simulink model "model_FOPTD_DMD_5SensorScenario_v1"  (R2021b)
settings: Solver=FixedStepAuto  StartTime=0.0  StopTime=20  FixedStep=TsSystem  MaxStep=0.01  RelTol=1e-3
values from neighbouring files (symbols this model uses):
  da = 0    [runSimulation_v1.m]
  ds = numSim    [runSimulation_v1.m]
  K = 1    [runSimulation_v1.m]
  Ka = 0    [runSimulation_v1.m]
  Ks = 0    [runSimulation_v1.m]
  L = 1    [runSimulation_v1.m]
  T = 0.1    [runSimulation_v1.m]
  TsSystem = 0.01    [runSimulation_v1.m]
libraries: simulink x2, slpidlib x1
settings Model: Creator=ahmet  LastModifiedBy=ahmet
settings SolverCC: AlgebraicLoopSolver=TrustRegion
settings DebuggingCC: SFMachineParentedDataDiag=warning

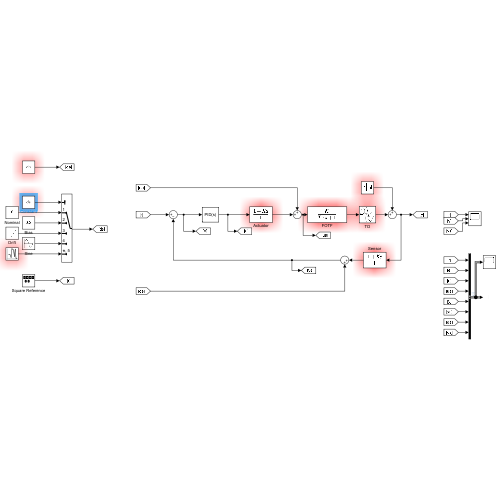
[thumbnail: Simulink's stored preview of the top-level diagram]
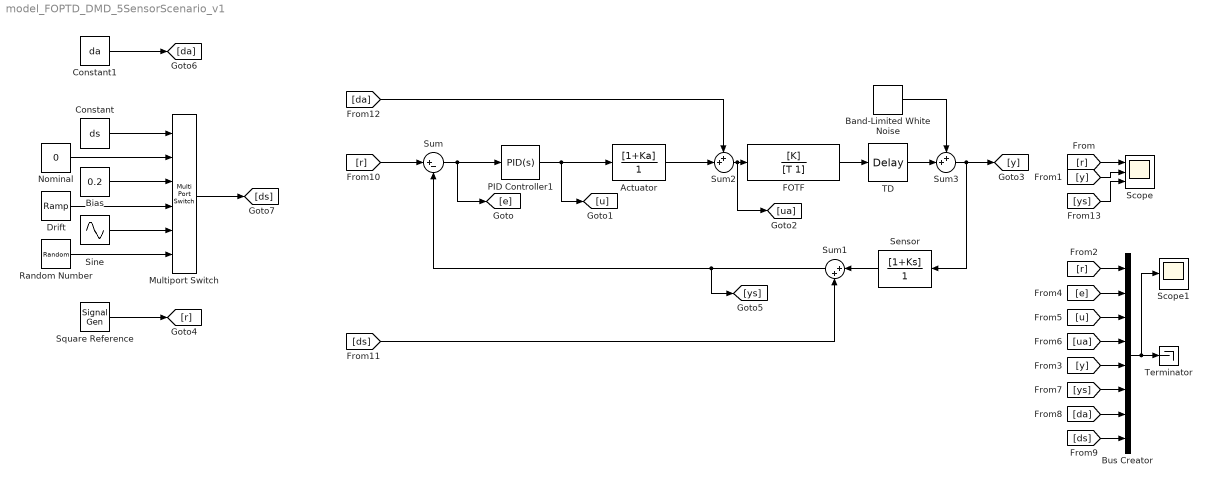
== system model_FOPTD_DMD_5SensorScenario_v1 ==
  Actuator : TransferFcn  Numerator=[1+Ka]  Denominator=[1]
  Band-Limited White Noise : simulink/Sources/Band-Limited White Noise  Cov=[1e-3*TsSystem]  Ts=TsSystem  seed=[23412+randi([-1000 1000],1,1)]
  Bias : Constant  Value=0.2
  Bus Creator : BusCreator  Inputs=8
  Constant : Constant  Value=ds
  Constant1 : Constant  Value=da
  Drift : simulink/Sources/Ramp  slope=1/10  start=0  InitialOutput=0
  FOTF : TransferFcn  Numerator=[K]  Denominator=[T 1]
  Multiport Switch : MultiPortSwitch  Inputs=5
  Nominal : Constant  Value=0
  PID Controller1 : slpidlib/PID Controller  Controller=PID  Form=Parallel  TimeDomain=Continuous-time  UseExternalTs=off  SampleTime=-1  IntegratorMethod=Forward Euler  FilterMethod=Forward Euler  ControllerParametersSource=internal  P=0.729803170365411  I=5.5584620696197  D=-0.0108988562858943  UseFilter=on  N=6.11275606083774  TunerSelectOption=Transfer Function Based (PID Tuner App)  InitialConditionSource=internal  InitialConditionForIntegrator=0  InitialConditionForFilter=0  DifferentiatorICPrevScaledInput=0  ExternalReset=none  TrackingMode=off  Kt=1  LimitOutput=off  SatLimitsSource=internal  UpperSaturationLimit=inf  LowerSaturationLimit=-inf  LinearizeAsGain=on  AntiWindupMode=none  Kb=1  POutMin=[]  POutMax=[]  IOutMin=[]  IOutMax=[]  DOutMin=[]  DOutMax=[]  NOutMin=[]  NOutMax=[]  SumOutMin=[]  SumOutMax=[]  SaturationOutMin=[]  SaturationOutMax=[]  PParamMin=[]  PParamMax=[]  IParamMin=[]  IParamMax=[]  DParamMin=[]  DParamMax=[]  NParamMin=[]  NParamMax=[]  KbParamMin=[]  KbParamMax=[]  KtParamMin=[]  KtParamMax=[]  KbOutMin=[]  KbOutMax=[]  KtOutMin=[]  KtOutMax=[]  IntegratorOutMin=[]  IntegratorOutMax=[]  FilterOutMin=[]  FilterOutMax=[]  SumI1OutMin=[]  SumI1OutMax=[]  SumI2OutMin=[]  SumI2OutMax=[]  SumI3OutMin=[]  SumI3OutMax=[]  SumI4OutMin=[]  SumI4OutMax=[]  SumDOutMin=[]  SumDOutMax=[]  DifferentiatorOutMin=[]  DifferentiatorOutMax=[]  FilterDiffOutCoefMin=[]  FilterDiffOutCoefMax=[]  ReciprocalOutMin=[]  ReciprocalOutMax=[]  SumDenOutMin=[]  SumDenOutMax=[]  SumNumOutMin=[]  SumNumOutMax=[]  DivideOutMin=[]  DivideOutMax=[]  UdiffTsProdOutMin=[]  UdiffTsProdOutMax=[]  NTsProdOutMin=[]  NTsProdOutMax=[]  UintegralTsProdOutMin=[]  UintegralTsProdOutMax=[]  UngainTsProdOutMin=[]  UngainTsProdOutMax=[]  IntegratorContinuousStateAttributes=''  IntegratorStateMustResolveToSignalObject=off  IntegratorRTWStateStorageClass=Auto  FilterContinuousStateAttributes=''  FilterStateMustResolveToSignalObject=off  FilterRTWStateStorageClass=Auto  ParallelPVariant=InternalParameters  IdealPVariant=Disabled  IVariant=InternalParameters  DVariant=InternalParameters  IntegratorVariant=Continuous  SatVariant=Disabled  AWVariant=Passthrough  PCopyVariant=Disabled  TRVariant=Disabled  FdbkBlocksVariant=Forward  IdealPFdbkVariant=Disabled  SatFdbkVariant=Disabled  DerivativeFilterVariant=ContFilter  NVariant=InternalParameters  NCopyVariant=Disabled  FilterICVariant=InternalICsFilter  IntegratorICVariant=InternalICs  ExternalResetVariant=Disabled  TRSumVariant=Passthrough  SumFdbkVariant=Disabled  SumVariant=Sum_PID  TsampFilterVariant=InternalTs  TsampNgainVariant=Passthrough  TsampIntegralVariant=Passthrough  ExternalSaturationOutDataTypeStr=Inherit: Same as second input
  Random Number : RandomNumber  SampleTime=TsSystem
  Scope : Scope  NumInputPorts=3
  Scope1 : Scope
  Sensor : TransferFcn  Numerator=[1+Ks]  Denominator=[1]
  Sine : Sin  Amplitude=0.5  Frequency=2*pi  SampleTime=0
  Square Reference : SignalGenerator  WaveForm=square  Frequency=0.1
  Sum : Sum  Inputs=|+-
  Sum1 : Sum  Inputs=|++
  Sum2 : Sum  Inputs=++|
  Sum3 : Sum  Inputs=++|
  TD : TransportDelay  DelayTime=L
  Terminator : Terminator
  wires:
  FOTF/1 -> TD/1
  Sum/1 -> PID Controller1/1, [e]
  [r] -> Scope/1
  [y] -> Scope/2
  Sensor/1 -> Sum1/1
  Sum1/1 -> [ys], Sum/2
  [r] -> Bus Creator/1
  [e] -> Bus Creator/2
  [u] -> Bus Creator/3
  [ua] -> Bus Creator/4
  [y] -> Bus Creator/5
  [ys] -> Bus Creator/6
  Bus Creator/1 -> Scope1/1, Terminator/1
  PID Controller1/1 -> Actuator/1, [u]
  TD/1 -> Sum3/2
  Sum3/1 -> Sensor/1, [y]
  Band-Limited White Noise/1 -> Sum3/1
  [ds] -> Bus Creator/8
  [da] -> Bus Creator/7
  [r] -> Sum/1
  [ds] -> Sum1/2
  [da] -> Sum2/1
  Constant1/1 -> [da]
  Actuator/1 -> Sum2/2
  Sum2/1 -> [ua], FOTF/1
  Square Reference/1 -> [r]
  Constant/1 -> Multiport Switch/1
  Multiport Switch/1 -> [ds]
  Drift/1 -> Multiport Switch/4
  Bias/1 -> Multiport Switch/3
  Nominal/1 -> Multiport Switch/2
  Sine/1 -> Multiport Switch/5
  Random Number/1 -> Multiport Switch/6
  [ys] -> Scope/3
